simulink model "LookupTableDynamic_above"  (R2017b)
settings: Solver=FixedStepDiscrete  StartTime=0.0  StopTime=10.0  FixedStep=0.200000  RelTol=1e-3  EnableMultiTasking=on
libraries: simulink x1
settings Model: Creator=hbourbou  LastModifiedBy=hbourbou
settings DataIOCC: LimitDataPoints=on  SaveFormat=StructureWithTime
settings OptimizationCC: LifeSpan=inf
settings DebuggingCC: SFUnexpectedBacktrackingDiag=warning  SFNoUnconditionalDefaultTransitionDiag=warning  SFExecutionAtInitializationDiag=none
settings HardwareCC: ProdBitPerSizeT=32  ProdBitPerPtrDiffT=32  ProdWordSize=32  ProdHWDeviceType=Specified
settings ModelReferenceCC: PropagateSignalLabelsOutOfModel=off
settings CodeAppCC: StateflowObjectComments=on
settings GRTTargetCC: TargetLangStandard=C89/C90 (ANSI)
settings ConfigComp: CovMetricSettings=dw  CovHtmlReporting=on  CovSaveCumulativeToWorkspaceVar=on  CovSaveSingleToWorkspaceVar=on  CovExternalEMLEnable=off

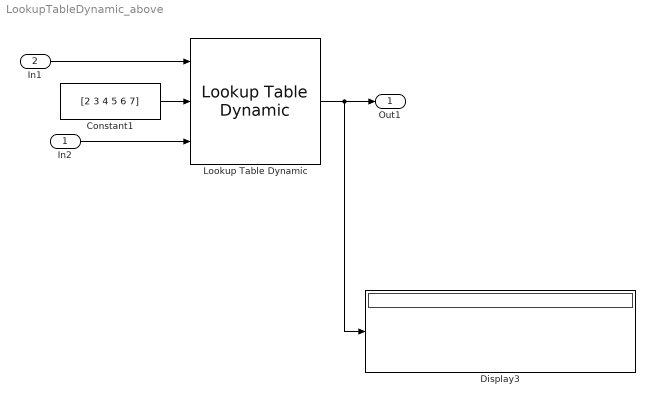
== system LookupTableDynamic_above ==
  In2 : Inport  PortDimensions=6
  In1 : Inport  Port=2  OutMin=-1  OutMax=10  PortDimensions=2
  Constant1 : Constant  Value=[2 3 4 5 6 7]
  Display3 : Display
  Lookup Table Dynamic : simulink/Lookup Tables/Lookup Table Dynamic  LookUpMeth=Use Input Above  OutDataType=fixdt('double')  OutScaling=[]  OutputDataTypeScalingMode=Specify via dialog  OutDataTypeStr=fixdt('double')  DoSatur=off
      settings: SourceProductName=Simulink
  Out1 : Outport
  wires:
  Lookup Table Dynamic/1 -> Display3/1, Out1/1
  In1/1 -> Lookup Table Dynamic/1
  Constant1/1 -> Lookup Table Dynamic/2
  In2/1 -> Lookup Table Dynamic/3
